simulink model "cascade"  (R2020b)
settings: Solver=VariableStepAuto  StartTime=0.0  StopTime=10.0  RelTol=1e-3
model workspace (MAT data in the model file):
  a = Simulink.Parameter
  a.Value = 1
  a.DataType = 'auto'
  a.Dimensions = [1 1]
  b = Simulink.Parameter
  b.Value = 1
  b.DataType = 'auto'
  b.Dimensions = [1 1]
  c = Simulink.Parameter
  c.Value = 2
  c.DataType = 'auto'
  c.Dimensions = [1 1]
  d = Simulink.Parameter
  d.Value = 1
  d.DataType = 'auto'
  d.Dimensions = [1 1]
  e = Simulink.Parameter
  e.Value = -1
  e.DataType = 'auto'
  e.Dimensions = [1 1]
  f = Simulink.Parameter
  f.Value = -1
  f.DataType = 'auto'
  f.Dimensions = [1 1]
settings Model: Creator=sushma  LastModifiedBy=sushma

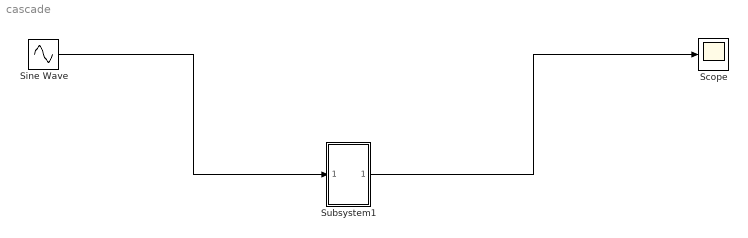
== system cascade ==
  Scope : Scope
  Sine Wave : Sin  SampleTime=0
  Subsystem1 : ModelReference  ModelNameDialog=Subsystem10  SimulationMode=Normal  ModelReferenceVersion=1.2
  wires:
  Sine Wave/1 -> Subsystem1/1
  Subsystem1/1 -> Scope/1
